simulink model "ModeloLineal"  (R2024b)
settings: Solver=VariableStepAuto  StartTime=0.0  StopTime=30  RelTol=1e-3
values from neighbouring files (symbols this model uses):
  Bs = 1200    [ValoresIniciales.m]
  Bt = 10    [ValoresIniciales.m]
  Fs = 0    [ValoresIniciales.m]
  Ks = 16000    [ValoresIniciales.m]    (also in quarter_car_model.m = 48000)
  Kt = 160000    [ValoresIniciales.m]    (also in quarter_car_model.m = 200000)
  Mb = 300    [ValoresIniciales.m]
  Mw = 30    [ValoresIniciales.m]
settings Model: Creator=juanp  LastModifiedBy=juanp

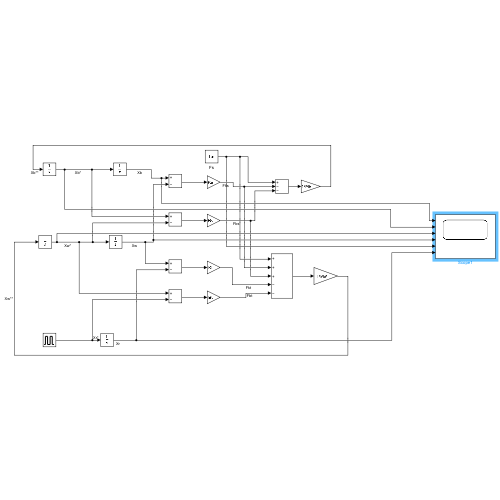
[thumbnail: Simulink's stored preview of the top-level diagram]
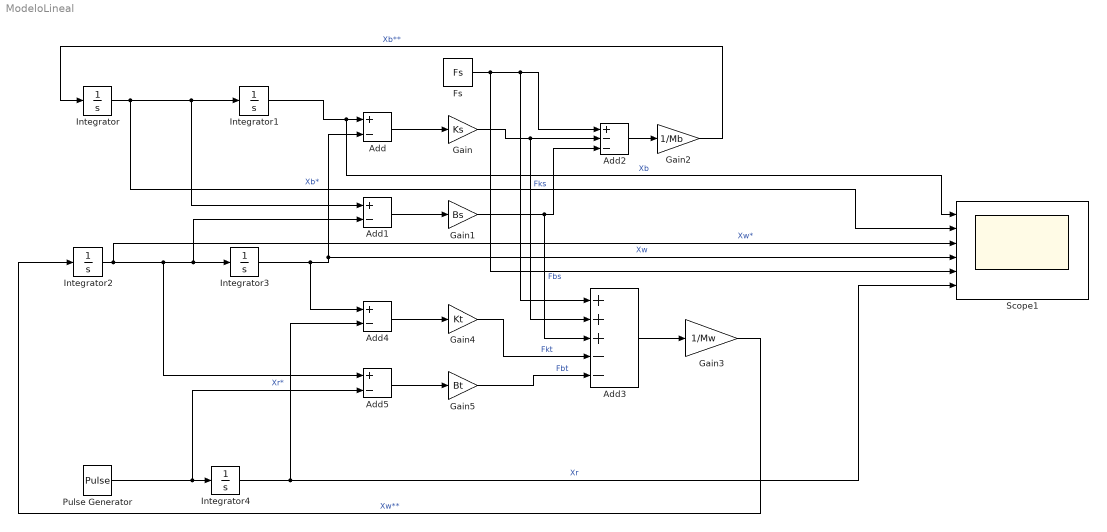
== system ModeloLineal ==
  Add{,1,4..5} (4 alike) : Sum  Inputs=+-
  Add2 : Sum  Inputs=+--
  Add3 : Sum  Inputs=+++--
  Fs : Constant  Value=Fs
  Gain : Gain  Gain=Ks
  Gain1 : Gain  Gain=Bs
  Gain2 : Gain  Gain=1/Mb
  Gain3 : Gain  Gain=1/Mw
  Gain4 : Gain  Gain=Kt
  Gain5 : Gain  Gain=Bt
  Integrator{,1..4} (5 alike) : Integrator
  Pulse Generator : DiscretePulseGenerator  PulseType=Time based  Amplitude=200  Period=10
  Scope1 : Scope  NumInputPorts=6
  wires:
  Integrator/1 -> Scope1/2, Add1/1, Integrator1/1  "Xb*"
  Gain2/1 -> Integrator/1  "Xb**"
  Integrator1/1 -> Scope1/1, Add/1  "Xb"
  Gain3/1 -> Integrator2/1  "Xw**"
  Integrator2/1 -> Scope1/3, Add5/1, Add1/2, Integrator3/1  "Xw*"
  Integrator3/1 -> Add4/1, Add/2, Scope1/4  "Xw"
  Add/1 -> Gain/1
  Gain/1 -> Add3/2, Add2/2  "Fks"
  Add1/1 -> Gain1/1
  Gain1/1 -> Add3/3, Add2/3  "Fbs"
  Fs/1 -> Scope1/5, Add3/1, Add2/1
  Add2/1 -> Gain2/1
  Pulse Generator/1 -> Add5/2, Integrator4/1  "Xr*"
  Add3/1 -> Gain3/1
  Add4/1 -> Gain4/1
  Gain4/1 -> Add3/4  "Fkt"
  Add5/1 -> Gain5/1
  Gain5/1 -> Add3/5  "Fbt"
  Integrator4/1 -> Add4/2, Scope1/6  "Xr"
